simulink model "heli"  (R2023b)
settings: Solver=FixedStepAuto  StartTime=0  StopTime=Ts  FixedStep=0.0025  MaxStep=0.01  RelTol=1e-3  AbsTol=1e-3
undefined symbols (not defined in the file): h, I, ic_euler_ang
libraries: simulink_extras x12, matrix_library x9, AP_Conector x2, shared6dof x1, aerolibobsolete x1
settings Model: Creator=FlightSim2  LastModifiedBy=okmatteson
settings SolverCC: AutoScaleAbsTol=off  AlgebraicLoopSolver=TrustRegion
settings DataIOCC: SaveFormat=Array  SaveOutput=off  SaveTime=off  ReturnWorkspaceOutputs=off
settings OptimizationCC: BlockReduction=off  BooleanDataType=off  ExpressionDepthLimit=2147483647  InitFltsAndDblsToZero=on  LifeSpan=inf
settings DebuggingCC: AlgebraicLoopMsg=none  SaveWithParameterizedLinksMsg=none  MergeDetectMultiDrivingBlocksExec=none  SignalResolutionControl=TryResolveAllWithWarning  InheritedTsInSrcMsg=none  MultiTaskDSMMsg=warning  MultiTaskCondExecSysMsg=none  FcnCallInpInsideContextMsg=warning  AllowSymbolicDim=off  UnknownTsInhSupMsg=none  StateNameClashWarn=warning  SFUnexpectedBacktrackingDiag=warning  SFNoUnconditionalDefaultTransitionDiag=warning  SFExecutionAtInitializationDiag=none  ArithmeticOperatorsInVariantConditions=warning
settings HardwareCC: ProdBitPerPointer=32  ProdBitPerSizeT=32  ProdBitPerPtrDiffT=32  ProdLargestAtomicFloat=None  ProdIntDivRoundTo=Undefined  ProdEndianess=Unspecified  ProdWordSize=32  ProdHWDeviceType=32-bit Generic  TargetUnknown=on
settings ModelReferenceCC: EnableRefExpFcnMdlSchedulingChecks=on  PropagateSignalLabelsOutOfModel=off
settings SFSimCC: SimUseLocalCustomCode=off  CustomCodeUndefinedFunction=UseInterfaceOnly
settings RTWCC: TemplateMakefile=grt_unix.tmf  RTWUseLocalCustomCode=off
settings CodeAppCC: StateflowObjectComments=on
settings GRTTargetCC: TargetFcnLib=ansi_tfl_tmw.mat  TargetLangStandard=C89/C90 (ANSI)  CombineOutputUpdateFcns=off  GRTInterface=on
settings ConfigComp: CovMetricSettings=dw  CovSaveCumulativeToWorkspaceVar=on  CovSaveSingleToWorkspaceVar=on  CovExternalEMLEnable=off

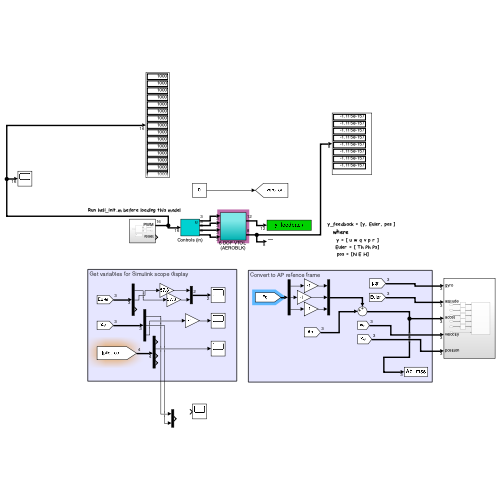
[thumbnail: Simulink's stored preview of the top-level diagram]
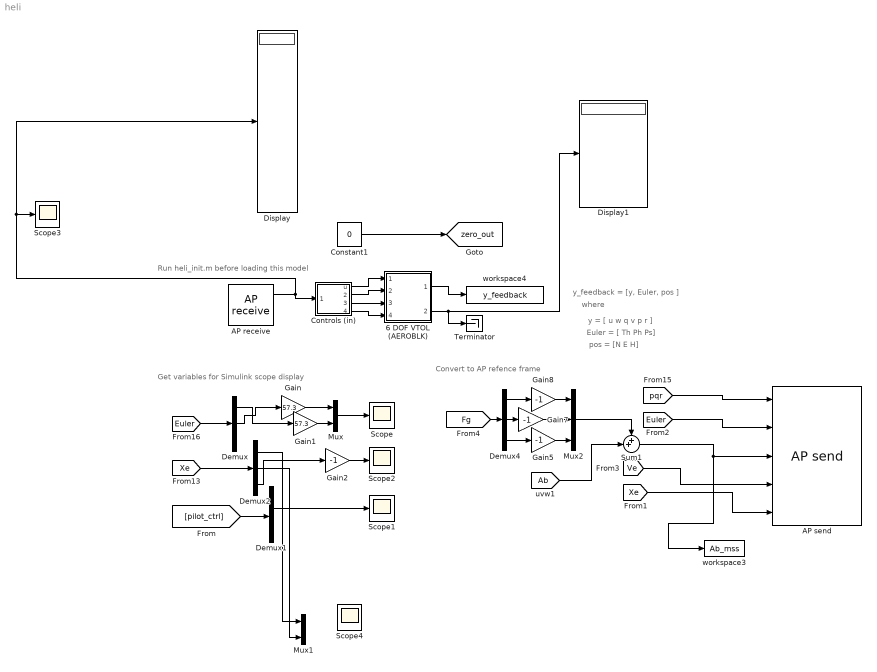
== system heli ==
  note: Run heli_init.m before loading this model
  note: Convert to AP refence frame
  note: Get variables for Simulink scope display
  note: y_feedback = [y, Euler, pos ]
  note: pos = [N E H]
  note: Euler = [ Th Ph Ps]
  note: y = [ u w q v p r ]
  note: where
  6 DOF VTOL (AEROBLK) : Subsystem
  AP receive : AP_Conector/AP receive  SystemSampleTime=-1  VariantActivationTime=update diagram  AllowFlexibleInterface=on  Latency=0  AutoFrameSizeCalculation=off
  AP send : AP_Conector/AP send  SystemSampleTime=-1  VariantActivationTime=update diagram  AllowFlexibleInterface=on  Latency=0  AutoFrameSizeCalculation=off
  Constant1 : Constant  Value=0
  Controls (in) : Subsystem
      mask Display: port_label('output',1,'u','texmode','on');
  Demux : Demux  Outputs=3
  Demux1 : Demux
  Demux2 : Demux  Outputs=3
  Demux4 : Demux  Outputs=3
  Display : Display
  Display1 : Display
  Gain : Gain  Gain=57.3
  Gain1 : Gain  Gain=57.3
  Gain{2,5,7..8} (4 alike) : Gain  Gain=-1
  Mux : Mux  Inputs=2
  Mux1 : Mux  Inputs=2
  Mux2 : Mux  Inputs=3
  Scope{,1..4} (5 alike) : Scope
  Sum1 : Sum  Inputs=++|
  Terminator : Terminator
  workspace3 : ToWorkspace  VariableName=Ab_mss
      settings: MaxDataPoints=max_saved
  workspace4 : ToWorkspace  VariableName=y_feedback
      settings: MaxDataPoints=max_saved
  tag scope: zero_out=global
  wires:
  Controls (in)/1(u) -> 6 DOF VTOL (AEROBLK)/1(Control1)
  6 DOF VTOL (AEROBLK)/1(Out1) -> workspace4/1
  [Euler] -> Demux/1
  Demux/1 -> Gain1/1
  Demux/2 -> Gain/1
  Mux/1 -> Scope/1
  [pilot_ctrl] -> Demux1/1
  Demux1/2 -> Scope1/1
  [Xe] -> Demux2/1
  Demux2/3 -> Gain2/1
  Gain/1 -> Mux/1
  Gain1/1 -> Mux/2
  Gain2/1 -> Scope2/1
  [pqr] -> AP send/1
  [Euler] -> AP send/2
  [Ve] -> AP send/4
  [Xe] -> AP send/5
  [Ab] -> Sum1/2
  [Fg] -> Demux4/1
  Demux4/1 -> Gain8/1
  Demux4/2 -> Gain7/1
  Mux2/1 -> Sum1/1
  Gain5/1 -> Mux2/3
  Demux4/3 -> Gain5/1
  Sum1/1 -> workspace3/1, AP send/3
  Gain8/1 -> Mux2/1
  Gain7/1 -> Mux2/2
  Constant1/1 -> [zero_out]
  Controls (in)/2(Outport) -> 6 DOF VTOL (AEROBLK)/2(Input)
  Controls (in)/3(Outport1) -> 6 DOF VTOL (AEROBLK)/3(Input1)
  Controls (in)/4(Outport2) -> 6 DOF VTOL (AEROBLK)/4(Input2)
  AP receive/1 -> Controls (in)/1(In1), Scope3/1, Display/1
  6 DOF VTOL (AEROBLK)/2(Outport) -> Terminator/1, Display1/1
  Demux2/1 -> Mux1/1
  Demux2/2 -> Mux1/2

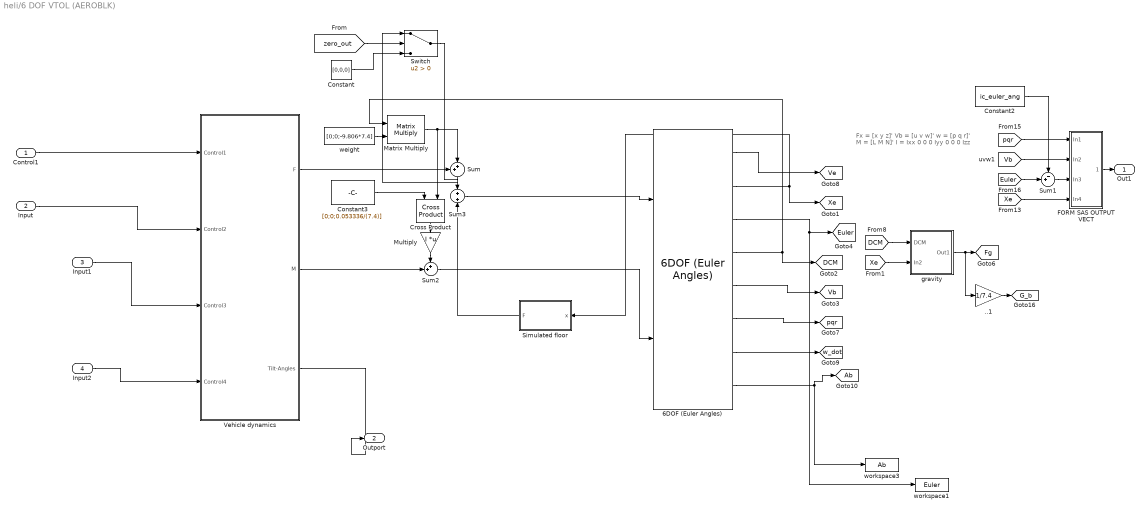
== system heli/6 DOF VTOL (AEROBLK) ==
  note: Fx = [x y z]'
      |
      | Vb = [u v w]'
      |
      | w = [p q r]'
      |
      | M = [L M N]'
      |
      | I =  Ixx  0     0
      |      0   Iyy    0
      |        	  0   0    Izz
  Control1 : Inport
  Input : Inport  Port=2
  Input1 : Inport  Port=3
  Input2 : Inport  Port=4
  ..1 : Gain  Gain=1/7.4  SaturateOnIntegerOverflow=on  OutDataTypeStr=Inherit: Same as input  ParamDataTypeStr=Inherit: Same as input
  6DOF (Euler Angles) : shared6dof/6DOF (Euler Angles)  units=Metric (MKS)  mtype=Fixed  rep=Euler Angles  xme_0=[0 0 0]  Vm_0=[0 0 0]  eul_0=[0 0 0]  pm_0=[0 0 0]  mass_0=7.4  mass_e=0.5  mass_f=2.0  inertia=I  inertia_e=eye(3)  inertia_f=2*eye(3)  k_quat=1.0  vre_flag=on  abi_flag=off  aMode=0  xme_statename=''  Vm_statename=''  eul_statename=''  quat_statename=''  pm_statename=''  mass_statename=''
  Constant : Constant  Value=[0,0,0]
  Constant2 : Constant  Value=ic_euler_ang
  Constant3 : Constant  Value=[0;0;0.053336/(7.4)]
  Cross Product : matrix_library/Cross Product
  FORM SAS OUTPUT VECT : Subsystem
      mask Display:
      | port_label('input',1,'pqr','texmode','on');
      | port_label('input',2,'Vb','texmode','on');
      | port_label('input',3,'Euler','texmode','on');
      | port_label('input',4,'Xe','texmode','on');
      | port_label('output',1,'y','texmode','on');
  Matrix Multiply : Product  Multiplication=Matrix(*)
  Multiply : Gain  Gain=I  Multiplication=Matrix(K*u)
  Simulated floor : MATLAB Function  TreatAsAtomicUnit=on  mask{x1=[-100; -0.1], x2=[100; -0.1], E=1000000, thickness=0.1, A=0.5^2}
  Sum : Sum  Inputs=++|
  Sum1 : Sum  Inputs=-+|
  Sum2 : Sum  Inputs=++|
  Sum3 : Sum  Inputs=+|+
  Switch : Switch  Criteria=u2 > Threshold  SaturateOnIntegerOverflow=off  InputSameDT=off
  Vehicle dynamics : Subsystem
  gravity : Subsystem
      mask Display:
      | port_label('input',1,'DCM','texmode','on');
      | port_label('input',2,'Xe','texmode','on');
      | port_label('output',1,'Fg','texmode','on');
  weight : Constant  Value=[0;0;-9.806*7.4]
  workspace1 : ToWorkspace  VariableName=Euler
      settings: MaxDataPoints=max_saved
  workspace3 : ToWorkspace  VariableName=Ab
      settings: MaxDataPoints=max_saved
  Out1 : Outport  VectorParamsAs1DForOutWhenUnconnected=off
  Outport : Outport  Port=2
  tag scope: Ab=global, DCM=global, Euler=global, Fg=global, G_b=global, Vb=global, Ve=global, Xe=global, pqr=global, w_dot=global
  wires:
  Control1/1 -> Vehicle dynamics/1(Control1)
  [pqr] -> FORM SAS OUTPUT VECT/1(In1)
  [Vb] -> FORM SAS OUTPUT VECT/2(In2)
  [Xe] -> FORM SAS OUTPUT VECT/4(In4)
  FORM SAS OUTPUT VECT/1(Out1) -> Out1/1
  6DOF (Euler Angles)/1 -> [Ve]
  6DOF (Euler Angles)/2 -> [Xe], Simulated floor/1(x)
  6DOF (Euler Angles)/4 -> [DCM], Matrix Multiply/1
  6DOF (Euler Angles)/5 -> [Vb]
  6DOF (Euler Angles)/6 -> [pqr]
  6DOF (Euler Angles)/7 -> [w_dot]
  6DOF (Euler Angles)/8 -> [Ab], workspace3/1
  Sum1/1 -> FORM SAS OUTPUT VECT/3(In3)
  gravity/1(Out1) -> ..1/1, [Fg]
  [Xe] -> gravity/2(In2)
  [DCM] -> gravity/1(DCM)
  ..1/1 -> [G_b]
  Constant2/1 -> Sum1/1
  [Euler] -> Sum1/2
  Input/1 -> Vehicle dynamics/2(Control2)
  Input1/1 -> Vehicle dynamics/3(Control3)
  Input2/1 -> Vehicle dynamics/4(Control4)
  Multiply/1 -> Sum2/1
  Cross Product/1 -> Multiply/1
  Vehicle dynamics/2(M) -> Sum2/2
  Constant3/1 -> Cross Product/1
  Sum2/1 -> 6DOF (Euler Angles)/2
  Sum3/1 -> 6DOF (Euler Angles)/1
  Matrix Multiply/1 -> Cross Product/2, Sum/2
  weight/1 -> Matrix Multiply/2
  6DOF (Euler Angles)/3 -> workspace1/1, [Euler]
  Simulated floor/1(F) -> Sum3/2
  Vehicle dynamics/1(F) -> Sum/1
  Switch/1 -> Sum3/1
  Constant/1 -> Switch/3
  Sum/1 -> Switch/1
  [zero_out] -> Switch/2
  Vehicle dynamics/3(Tilt-Angles) -> Outport/1

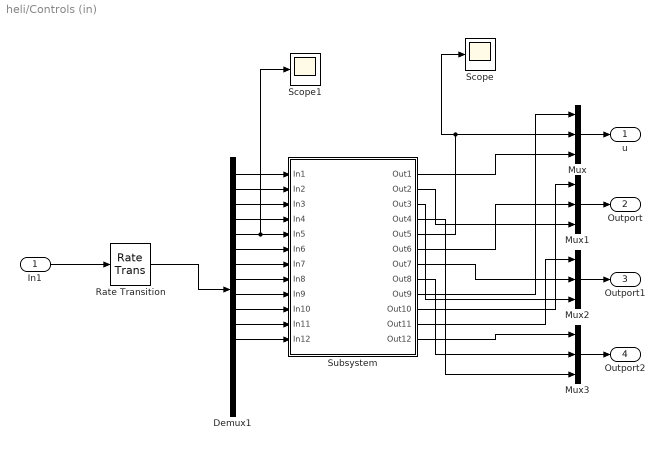
== system heli/Controls (in) ==
  In1 : Inport
  Demux1 : Demux  Outputs=16
  Mux{,1..3} (4 alike) : Mux  Inputs=3
  Rate Transition : RateTransition
  Scope : Scope
  Scope1 : Scope
  Subsystem : Subsystem
  u : Outport  VectorParamsAs1DForOutWhenUnconnected=off
  Outport : Outport  Port=2
  Outport1 : Outport  Port=3
  Outport2 : Outport  Port=4
  wires:
  In1/1 -> Rate Transition/1
  Subsystem/1(Out1) -> Mux/3
  Rate Transition/1 -> Demux1/1
  Demux1/2 -> Subsystem/2(In2)
  Demux1/7 -> Subsystem/7(In7)
  Subsystem/9(Out9) -> Mux/1
  Mux/1 -> u/1
  Demux1/12 -> Subsystem/12(In12)
  Demux1/10 -> Subsystem/10(In10)
  Subsystem/6(Out6) -> Mux1/2
  Demux1/6 -> Subsystem/6(In6)
  Subsystem/12(Out12) -> Mux3/1
  Subsystem/2(Out2) -> Mux1/3
  Subsystem/10(Out10) -> Mux1/1
  Subsystem/11(Out11) -> Mux2/1
  Demux1/9 -> Subsystem/9(In9)
  Subsystem/4(Out4) -> Mux3/3
  Mux1/1 -> Outport/1
  Subsystem/8(Out8) -> Mux3/2
  Subsystem/5(Out5) -> Mux/2, Scope/1
  Demux1/4 -> Subsystem/4(In4)
  Subsystem/7(Out7) -> Mux2/2
  Mux2/1 -> Outport1/1
  Mux3/1 -> Outport2/1
  Demux1/11 -> Subsystem/11(In11)
  Demux1/5 -> Scope1/1, Subsystem/5(In5)
  Demux1/8 -> Subsystem/8(In8)
  Subsystem/3(Out3) -> Mux2/3
  Demux1/1 -> Subsystem/1(In1)
  Demux1/3 -> Subsystem/3(In3)

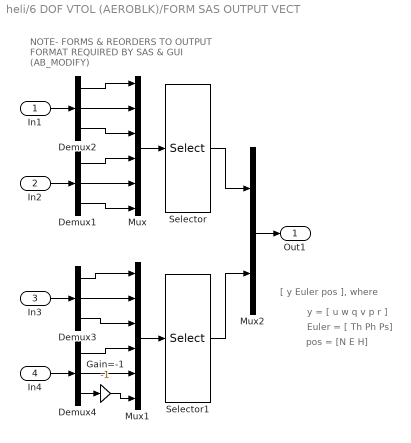
== system heli/6 DOF VTOL (AEROBLK)/FORM SAS OUTPUT VECT ==
  note: NOTE- FORMS & REORDERS TO OUTPUT FORMAT
      | REQUIRED BY SAS & GUI (AB_MODIFY)
  note: [ y Euler pos ], where
  note: pos = [N E H]
  note: Euler = [ Th Ph Ps]
  note: y = [ u w q v p r ]
  In1 : Inport
  In2 : Inport  Port=2
  In3 : Inport  Port=3
  In4 : Inport  Port=4
  Demux{1..4} (4 alike) : Demux  Outputs=3
  Gain=-1 : Gain  Gain=-1
  Mux : Mux  Inputs=6
  Mux1 : Mux  Inputs=6
  Mux2 : Mux  Inputs=2
  Selector : Selector  InputPortWidth=6  IndexOptions=Index vector (dialog)  Indices=[4 6 2 5 1 3]  OutputSizes=1
  Selector1 : Selector  InputPortWidth=6  IndexOptions=Index vector (dialog)  Indices=[2 1 3 4 5 6]  OutputSizes=1
  Out1 : Outport  VectorParamsAs1DForOutWhenUnconnected=off
  wires:
  Demux2/1 -> Mux/1
  Demux2/2 -> Mux/2
  Demux1/1 -> Mux/4
  Demux1/2 -> Mux/5
  Demux1/3 -> Mux/6
  Mux/1 -> Selector/1
  Demux2/3 -> Mux/3
  Mux1/1 -> Selector1/1
  Selector/1 -> Mux2/1
  Selector1/1 -> Mux2/2
  Demux3/1 -> Mux1/1
  Demux3/2 -> Mux1/2
  Demux3/3 -> Mux1/3
  Demux4/1 -> Mux1/4
  Demux4/2 -> Mux1/5
  Gain=-1/1 -> Mux1/6
  Demux4/3 -> Gain=-1/1
  In1/1 -> Demux2/1
  In2/1 -> Demux1/1
  Mux2/1 -> Out1/1
  In3/1 -> Demux3/1
  In4/1 -> Demux4/1

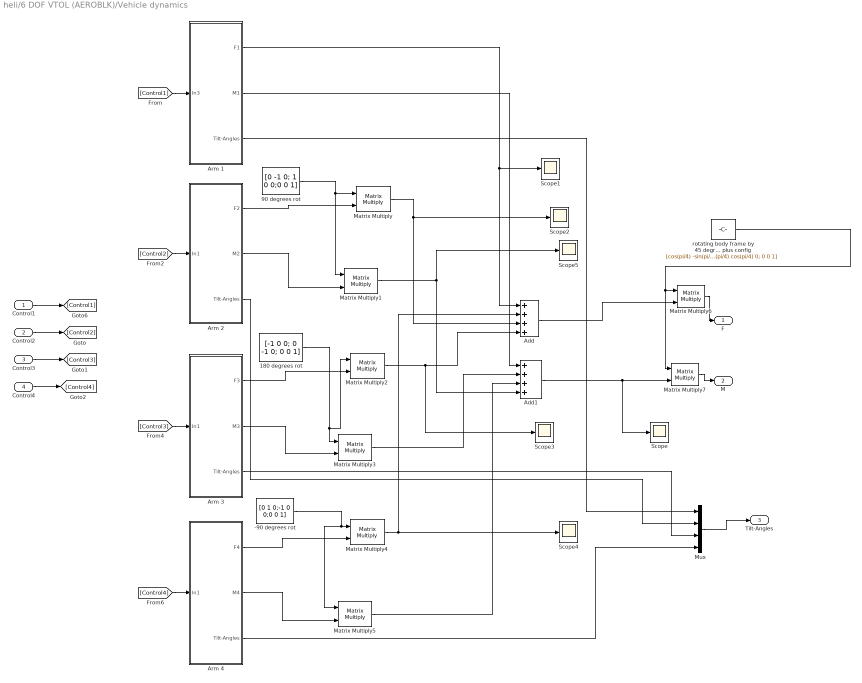
== system heli/6 DOF VTOL (AEROBLK)/Vehicle dynamics ==
  Control1 : Inport
  Control2 : Inport  Port=2
  Control3 : Inport  Port=3
  Control4 : Inport  Port=4
  -90 degrees rot : Constant  Value=[0 1 0;-1 0 0;0 0 1]
  180 degrees rot : Constant  Value=[-1 0 0; 0 -1 0; 0 0 1]
  90 degrees rot : Constant  Value=[0 -1 0; 1 0 0;0 0 1]
  Add : Sum  Inputs=++++
  Add1 : Sum  Inputs=++++
  Arm 1 : Subsystem
  Arm 2 : Subsystem
  Arm 3 : Subsystem
  Arm 4 : Subsystem
  Matrix Multiply{,1..7} (8 alike) : Product  Multiplication=Matrix(*)
  Mux : Mux
  Scope{,1..5} (6 alike) : Scope
  rotating body frame by 45 degrees to X config because vehicle dynamics was done in plus config : Constant  Value=|
      | [cos(pi/4) -sin(pi/4) 0;
      | sin(pi/4) cos(pi/4) 0;
      | 0 0 1]
  F : Outport
  M : Outport  Port=2
  Tilt-Angles : Outport  Port=3
  wires:
  Control1/1 -> [Control1]
  Control2/1 -> [Control2]
  Control3/1 -> [Control3]
  Control4/1 -> [Control4]
  [Control1] -> Arm 1/1(In3)
  Arm 1/1(F1) -> Add/1, Scope1/1
  Arm 1/2(M1) -> Add1/1
  90 degrees rot/1 -> Matrix Multiply1/1, Matrix Multiply/1
  Arm 2/1(F2) -> Matrix Multiply/2
  Matrix Multiply/1 -> Scope2/1, Add/3
  Arm 2/2(M2) -> Matrix Multiply1/2
  Matrix Multiply1/1 -> Add1/4, Scope5/1
  [Control2] -> Arm 2/1(In1)
  -90 degrees rot/1 -> Matrix Multiply5/1, Matrix Multiply4/1
  Arm 3/1(F3) -> Matrix Multiply2/2
  Matrix Multiply3/1 -> Add1/2
  [Control3] -> Arm 3/1(In1)
  Arm 3/2(M3) -> Matrix Multiply3/2
  180 degrees rot/1 -> Matrix Multiply3/1, Matrix Multiply2/1
  Arm 4/2(M4) -> Matrix Multiply5/2
  Arm 4/1(F4) -> Matrix Multiply4/2
  Matrix Multiply5/1 -> Add1/3
  [Control4] -> Arm 4/1(In1)
  Matrix Multiply2/1 -> Scope3/1, Add/4
  Matrix Multiply4/1 -> Add/2, Scope4/1
  rotating body frame by 45 degrees to X config because vehicle dynamics was done in plus config/1 -> Matrix Multiply6/1, Matrix Multiply7/1
  Add/1 -> Matrix Multiply6/2
  Add1/1 -> Matrix Multiply7/2, Scope/1
  Matrix Multiply7/1 -> M/1
  Matrix Multiply6/1 -> F/1
  Arm 1/3(Tilt-Angles) -> Mux/1
  Arm 2/3(Tilt-Angles) -> Mux/2
  Arm 3/3(Tilt-Angles) -> Mux/3
  Arm 4/3(Tilt-Angles) -> Mux/4
  Mux/1 -> Tilt-Angles/1

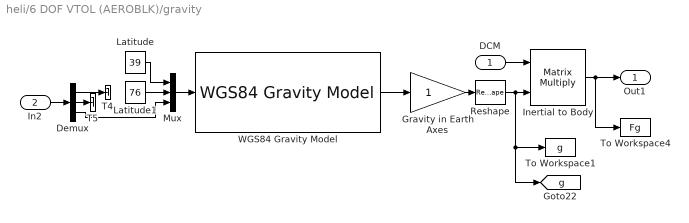
== system heli/6 DOF VTOL (AEROBLK)/gravity ==
  DCM : Inport
  In2 : Inport  Port=2
  Demux : Demux  Outputs=3
  Gravity in Earth Axes : Gain  SaturateOnIntegerOverflow=on  OutDataTypeStr=Inherit: Same as input  ParamDataTypeStr=Inherit: Same as input
  Inertial to Body : Product  Multiplication=Matrix(*)  InputSameDT=on  SaturateOnIntegerOverflow=on  OutDataTypeStr=Inherit: Same as first input
  Latitude : Constant  Value=39
  Latitude1 : Constant  Value=76
  Mux : Mux  Inputs=3
  Reshape : Reshape
  T4 : Terminator
  T5 : Terminator
  To Workspace1 : ToWorkspace  VariableName=g  SampleTime=-1
      settings: MaxDataPoints=max_saved
  To Workspace4 : ToWorkspace  VariableName=Fg  SampleTime=-1
      settings: MaxDataPoints=max_saved
  "WGS84 Gravity Model " : aerolibobsolete/WGS84 Gravity Model   model=WGS84 Exact  units=Metric (MKS)  no_atmos=on  precessing=on  jd_loc=off  month=October  day=10  year=2004  no_centrifugal=on  action=None
  Out1 : Outport  VectorParamsAs1DForOutWhenUnconnected=off
  tag scope: g=global
  wires:
  In2/1 -> Demux/1
  Demux/2 -> T5/1
  Demux/1 -> T4/1
  Inertial to Body/1 -> To Workspace4/1, Out1/1
  DCM/1 -> Inertial to Body/1
  Gravity in Earth Axes/1 -> Reshape/1
  "WGS84 Gravity Model "/1 -> Gravity in Earth Axes/1
  Mux/1 -> "WGS84 Gravity Model "/1
  Reshape/1 -> Inertial to Body/2, To Workspace1/1, [g]
  Latitude1/1 -> Mux/2
  Latitude/1 -> Mux/1
  Demux/3 -> Mux/3

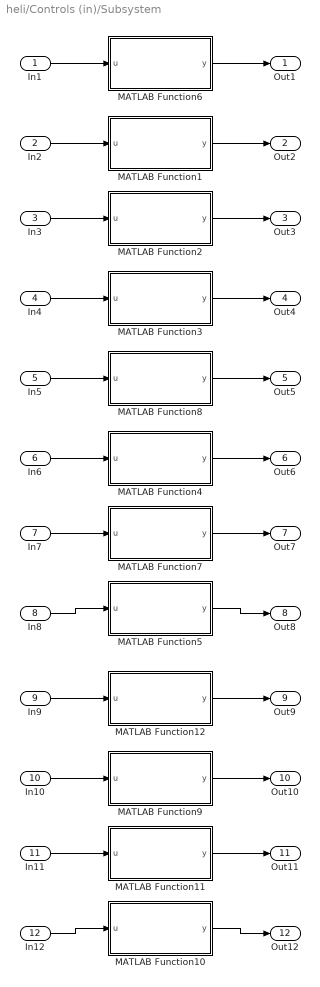
== system heli/Controls (in)/Subsystem ==
  In1 : Inport
  In2 : Inport  Port=2
  In3 : Inport  Port=3
  In4 : Inport  Port=4
  In5 : Inport  Port=5
  In6 : Inport  Port=6
  In7 : Inport  Port=7
  In8 : Inport  Port=8
  In9 : Inport  Port=9
  In10 : Inport  Port=10
  In11 : Inport  Port=11
  In12 : Inport  Port=12
  MATLAB Function1 : MATLAB Function  TreatAsAtomicUnit=on  mask{min_in=1000, min_out=0, max_in=2000, max_out=633}
  MATLAB Function10 : MATLAB Function  TreatAsAtomicUnit=on  mask{min_in=682, min_out=-1.57, max_in=2318, max_out=1.57}
  MATLAB Function11 : MATLAB Function  TreatAsAtomicUnit=on  mask{min_in=682, min_out=-1.57, max_in=2318, max_out=1.57}
  MATLAB Function12 : MATLAB Function  TreatAsAtomicUnit=on  mask{min_in=682, min_out=-1.57, max_in=2318, max_out=1.57}
  MATLAB Function2 : MATLAB Function  TreatAsAtomicUnit=on  mask{min_in=1000, min_out=0, max_in=2000, max_out=633}
  MATLAB Function3 : MATLAB Function  TreatAsAtomicUnit=on  mask{min_in=1000, min_out=0, max_in=2000, max_out=633}
  MATLAB Function4 : MATLAB Function  TreatAsAtomicUnit=on  mask{min_in=682, min_out=-1.57, max_in=2318, max_out=1.57}
  MATLAB Function5 : MATLAB Function  TreatAsAtomicUnit=on  mask{min_in=682, min_out=-1.57, max_in=2318, max_out=1.57}
  MATLAB Function6 : MATLAB Function  TreatAsAtomicUnit=on  mask{min_in=1000, min_out=0, max_in=2000, max_out=633}
  MATLAB Function7 : MATLAB Function  TreatAsAtomicUnit=on  mask{min_in=682, min_out=-1.57, max_in=2318, max_out=1.57}
  MATLAB Function8 : MATLAB Function  TreatAsAtomicUnit=on  mask{min_in=682, min_out=-1.57, max_in=2318, max_out=1.57}
  MATLAB Function9 : MATLAB Function  TreatAsAtomicUnit=on  mask{min_in=682, min_out=-1.57, max_in=2318, max_out=1.57}
  Out1 : Outport
  Out2 : Outport  Port=2
  Out3 : Outport  Port=3
  Out4 : Outport  Port=4
  Out5 : Outport  Port=5
  Out6 : Outport  Port=6
  Out7 : Outport  Port=7
  Out8 : Outport  Port=8
  Out9 : Outport  Port=9
  Out10 : Outport  Port=10
  Out11 : Outport  Port=11
  Out12 : Outport  Port=12
  wires:
  In1/1 -> MATLAB Function6/1(u)
  MATLAB Function6/1(y) -> Out1/1
  In2/1 -> MATLAB Function1/1(u)
  MATLAB Function1/1(y) -> Out2/1
  MATLAB Function2/1(y) -> Out3/1
  In3/1 -> MATLAB Function2/1(u)
  In4/1 -> MATLAB Function3/1(u)
  MATLAB Function3/1(y) -> Out4/1
  In5/1 -> MATLAB Function8/1(u)
  MATLAB Function8/1(y) -> Out5/1
  MATLAB Function4/1(y) -> Out6/1
  In6/1 -> MATLAB Function4/1(u)
  In7/1 -> MATLAB Function7/1(u)
  MATLAB Function7/1(y) -> Out7/1
  In8/1 -> MATLAB Function5/1(u)
  MATLAB Function5/1(y) -> Out8/1
  In9/1 -> MATLAB Function12/1(u)
  MATLAB Function12/1(y) -> Out9/1
  MATLAB Function9/1(y) -> Out10/1
  In10/1 -> MATLAB Function9/1(u)
  In11/1 -> MATLAB Function11/1(u)
  MATLAB Function11/1(y) -> Out11/1
  In12/1 -> MATLAB Function10/1(u)
  MATLAB Function10/1(y) -> Out12/1

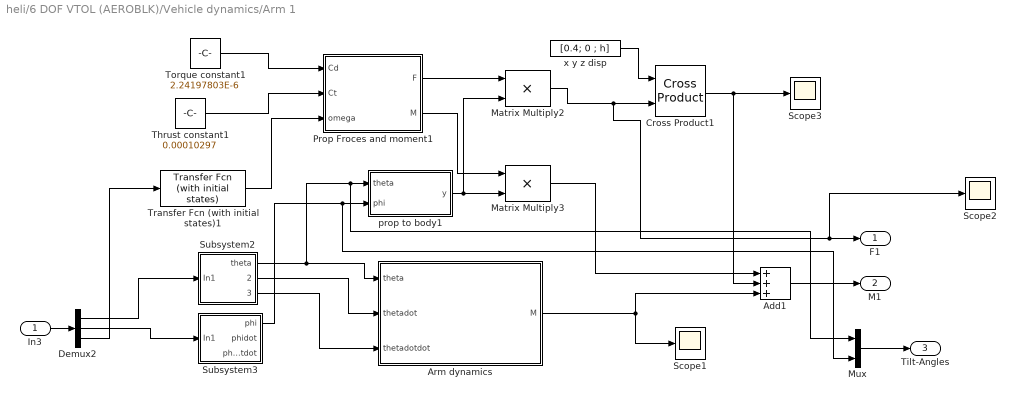
== system heli/6 DOF VTOL (AEROBLK)/Vehicle dynamics/Arm 1 ==
  In3 : Inport
  Add1 : Sum  Inputs=+++
  Arm dynamics : Subsystem
  Cross Product1 : matrix_library/Cross Product
  Demux2 : Demux  Outputs=3
  Matrix Multiply2 : Product
  Matrix Multiply3 : Product
  Mux : Mux  Inputs=2
  Prop Froces and moment1 : Subsystem
  Scope1 : Scope
  Scope2 : Scope
  Scope3 : Scope
  Subsystem2 : Subsystem
  Subsystem3 : Subsystem
  Thrust constant1 : Constant  Value=0.00010297
  Torque constant1 : Constant  Value=2.24197803E-6
  Transfer Fcn (with initial states)1 : simulink_extras/Additional Linear/Transfer Fcn (with initial states)  N=[153.35]  D=[1 20.06 153.35]  X0=0
  prop to body1 : MATLAB Function  TreatAsAtomicUnit=on
  x y z disp : Constant  Value=[0.4; 0 ; h]
  F1 : Outport
  M1 : Outport  Port=2
  Tilt-Angles : Outport  Port=3
  wires:
  x y z disp/1 -> Cross Product1/1
  Subsystem2/2(thetadot) -> Arm dynamics/2(thetadot)
  Cross Product1/1 -> Add1/2, Scope3/1
  In3/1 -> Demux2/1
  Prop Froces and moment1/1(F) -> Matrix Multiply2/1
  Arm dynamics/1(M) -> Add1/3, Scope1/1
  Demux2/2 -> Subsystem3/1(In1)
  Thrust constant1/1 -> Prop Froces and moment1/2(Ct)
  Torque constant1/1 -> Prop Froces and moment1/1(Cd)
  Add1/1 -> M1/1
  Matrix Multiply3/1 -> Add1/1
  prop to body1/1(y) -> Matrix Multiply3/2, Matrix Multiply2/2
  Prop Froces and moment1/2(M) -> Matrix Multiply3/1
  Demux2/1 -> Subsystem2/1(In1)
  Subsystem2/1(theta) -> Arm dynamics/1(theta), Mux/1, prop to body1/1(theta)
  Matrix Multiply2/1 -> Cross Product1/2, Scope2/1, F1/1
  Subsystem3/1(phi) -> Mux/2, prop to body1/2(phi)
  Subsystem2/3(thetadotdot) -> Arm dynamics/3(thetadotdot)
  Demux2/3 -> Transfer Fcn (with initial states)1/1
  Transfer Fcn (with initial states)1/1 -> Prop Froces and moment1/3(omega)
  Mux/1 -> Tilt-Angles/1

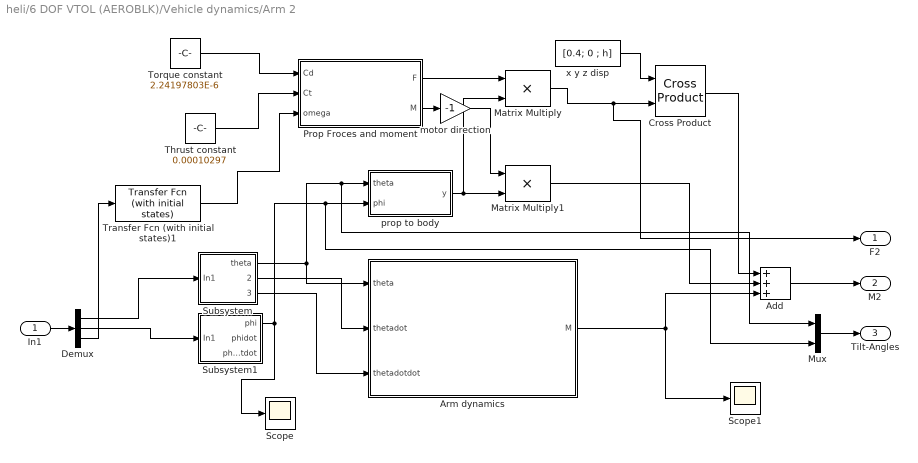
== system heli/6 DOF VTOL (AEROBLK)/Vehicle dynamics/Arm 2 ==
  In1 : Inport
  Add : Sum  Inputs=+++
  Arm dynamics : Subsystem
  Cross Product : matrix_library/Cross Product
  Demux : Demux  Outputs=3
  Matrix Multiply : Product
  Matrix Multiply1 : Product
  Mux : Mux  Inputs=2
  Prop Froces and moment : Subsystem
  Scope : Scope
  Scope1 : Scope
  Subsystem : Subsystem
  Subsystem1 : Subsystem
  Thrust constant : Constant  Value=0.00010297
  Torque constant : Constant  Value=2.24197803E-6
  Transfer Fcn (with initial states)1 : simulink_extras/Additional Linear/Transfer Fcn (with initial states)  N=[153.35]  D=[1 20.06 153.35]  X0=0
  motor direction : Gain  Gain=-1
  prop to body : MATLAB Function  TreatAsAtomicUnit=on
  x y z disp : Constant  Value=[0.4; 0 ; h]
  F2 : Outport
  M2 : Outport  Port=2
  Tilt-Angles : Outport  Port=3
  wires:
  prop to body/1(y) -> Matrix Multiply1/2, Matrix Multiply/2
  Demux/2 -> Subsystem1/1(In1)
  Matrix Multiply/1 -> Cross Product/2, F2/1
  Prop Froces and moment/1(F) -> Matrix Multiply/1
  Subsystem/1(theta) -> Arm dynamics/1(theta), Mux/1, prop to body/1(theta)
  Matrix Multiply1/1 -> Add/2
  Prop Froces and moment/2(M) -> motor direction/1
  Subsystem1/1(phi) -> Scope/1, Mux/2, prop to body/2(phi)
  Demux/1 -> Subsystem/1(In1)
  x y z disp/1 -> Cross Product/1
  Add/1 -> M2/1
  Torque constant/1 -> Prop Froces and moment/1(Cd)
  Thrust constant/1 -> Prop Froces and moment/2(Ct)
  Cross Product/1 -> Add/1
  In1/1 -> Demux/1
  Subsystem/2(thetadot) -> Arm dynamics/2(thetadot)
  Subsystem/3(thetadotdot) -> Arm dynamics/3(thetadotdot)
  Arm dynamics/1(M) -> Add/3, Scope1/1
  Demux/3 -> Transfer Fcn (with initial states)1/1
  motor direction/1 -> Matrix Multiply1/1
  Transfer Fcn (with initial states)1/1 -> Prop Froces and moment/3(omega)
  Mux/1 -> Tilt-Angles/1

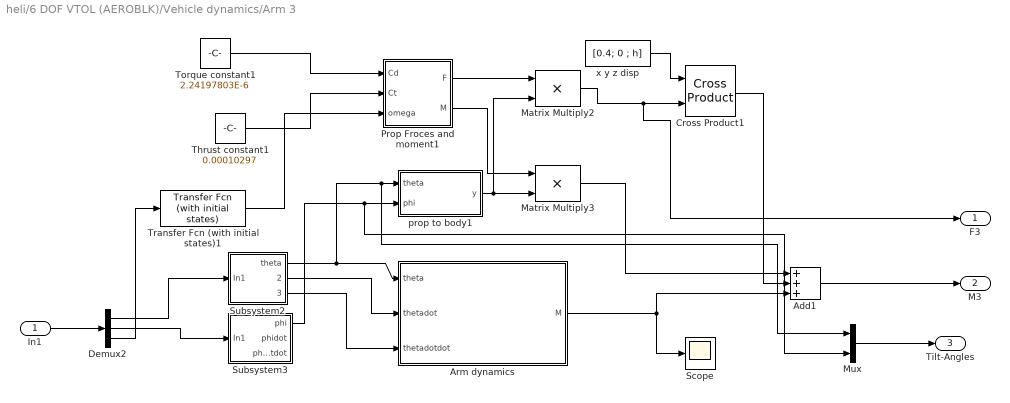
== system heli/6 DOF VTOL (AEROBLK)/Vehicle dynamics/Arm 3 ==
  In1 : Inport
  Add1 : Sum  Inputs=+++
  Arm dynamics : Subsystem
  Cross Product1 : matrix_library/Cross Product
  Demux2 : Demux  Outputs=3
  Matrix Multiply2 : Product
  Matrix Multiply3 : Product
  Mux : Mux  Inputs=2
  Prop Froces and moment1 : Subsystem
  Scope : Scope
  Subsystem2 : Subsystem
  Subsystem3 : Subsystem
  Thrust constant1 : Constant  Value=0.00010297
  Torque constant1 : Constant  Value=2.24197803E-6
  Transfer Fcn (with initial states)1 : simulink_extras/Additional Linear/Transfer Fcn (with initial states)  N=[153.35]  D=[1 20.06 153.35]  X0=0
  prop to body1 : MATLAB Function  TreatAsAtomicUnit=on
  x y z disp : Constant  Value=[0.4; 0 ; h]
  F3 : Outport
  M3 : Outport  Port=2
  Tilt-Angles : Outport  Port=3
  wires:
  x y z disp/1 -> Cross Product1/1
  Subsystem2/2(thetadot) -> Arm dynamics/2(thetadot)
  Cross Product1/1 -> Add1/2
  In1/1 -> Demux2/1
  Prop Froces and moment1/1(F) -> Matrix Multiply2/1
  Arm dynamics/1(M) -> Add1/3, Scope/1
  Demux2/2 -> Subsystem3/1(In1)
  Thrust constant1/1 -> Prop Froces and moment1/2(Ct)
  Torque constant1/1 -> Prop Froces and moment1/1(Cd)
  Add1/1 -> M3/1
  Matrix Multiply3/1 -> Add1/1
  prop to body1/1(y) -> Matrix Multiply3/2, Matrix Multiply2/2
  Prop Froces and moment1/2(M) -> Matrix Multiply3/1
  Demux2/1 -> Subsystem2/1(In1)
  Subsystem2/1(theta) -> Arm dynamics/1(theta), Mux/1, prop to body1/1(theta)
  Demux2/3 -> Transfer Fcn (with initial states)1/1
  Matrix Multiply2/1 -> Cross Product1/2, F3/1
  Subsystem3/1(phi) -> Mux/2, prop to body1/2(phi)
  Subsystem2/3(thetadotdot) -> Arm dynamics/3(thetadotdot)
  Transfer Fcn (with initial states)1/1 -> Prop Froces and moment1/3(omega)
  Mux/1 -> Tilt-Angles/1

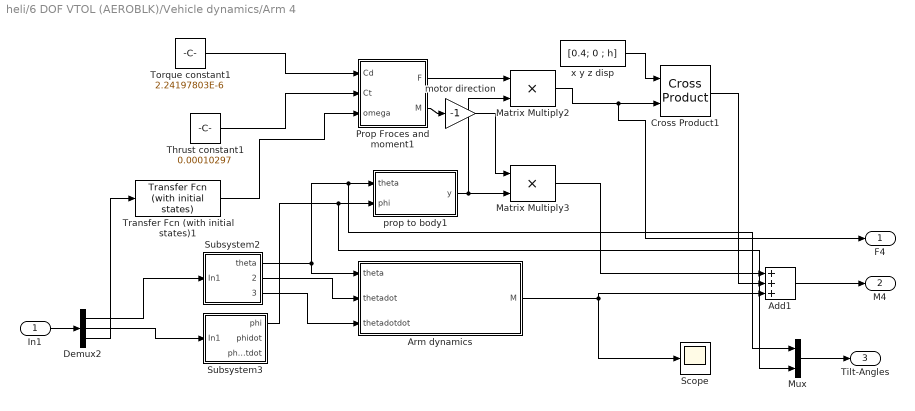
== system heli/6 DOF VTOL (AEROBLK)/Vehicle dynamics/Arm 4 ==
  In1 : Inport
  Add1 : Sum  Inputs=+++
  Arm dynamics : Subsystem
  Cross Product1 : matrix_library/Cross Product
  Demux2 : Demux  Outputs=3
  Matrix Multiply2 : Product
  Matrix Multiply3 : Product
  Mux : Mux  Inputs=2
  Prop Froces and moment1 : Subsystem
  Scope : Scope
  Subsystem2 : Subsystem
  Subsystem3 : Subsystem
  Thrust constant1 : Constant  Value=0.00010297
  Torque constant1 : Constant  Value=2.24197803E-6
  Transfer Fcn (with initial states)1 : simulink_extras/Additional Linear/Transfer Fcn (with initial states)  N=[153.35]  D=[1 20.06 153.35]  X0=0
  motor direction : Gain  Gain=-1
  prop to body1 : MATLAB Function  TreatAsAtomicUnit=on
  x y z disp : Constant  Value=[0.4; 0 ; h]
  F4 : Outport
  M4 : Outport  Port=2
  Tilt-Angles : Outport  Port=3
  wires:
  x y z disp/1 -> Cross Product1/1
  Subsystem2/2(thetadot) -> Arm dynamics/2(thetadot)
  Cross Product1/1 -> Add1/2
  In1/1 -> Demux2/1
  Prop Froces and moment1/1(F) -> Matrix Multiply2/1
  Arm dynamics/1(M) -> Add1/3, Scope/1
  Demux2/2 -> Subsystem3/1(In1)
  Thrust constant1/1 -> Prop Froces and moment1/2(Ct)
  Torque constant1/1 -> Prop Froces and moment1/1(Cd)
  Add1/1 -> M4/1
  Matrix Multiply3/1 -> Add1/1
  prop to body1/1(y) -> Matrix Multiply3/2, Matrix Multiply2/2
  Prop Froces and moment1/2(M) -> motor direction/1
  Demux2/1 -> Subsystem2/1(In1)
  Subsystem2/1(theta) -> Arm dynamics/1(theta), Mux/1, prop to body1/1(theta)
  Matrix Multiply2/1 -> Cross Product1/2, F4/1
  Subsystem3/1(phi) -> Mux/2, prop to body1/2(phi)
  Subsystem2/3(thetadotdot) -> Arm dynamics/3(thetadotdot)
  Demux2/3 -> Transfer Fcn (with initial states)1/1
  motor direction/1 -> Matrix Multiply3/1
  Transfer Fcn (with initial states)1/1 -> Prop Froces and moment1/3(omega)
  Mux/1 -> Tilt-Angles/1

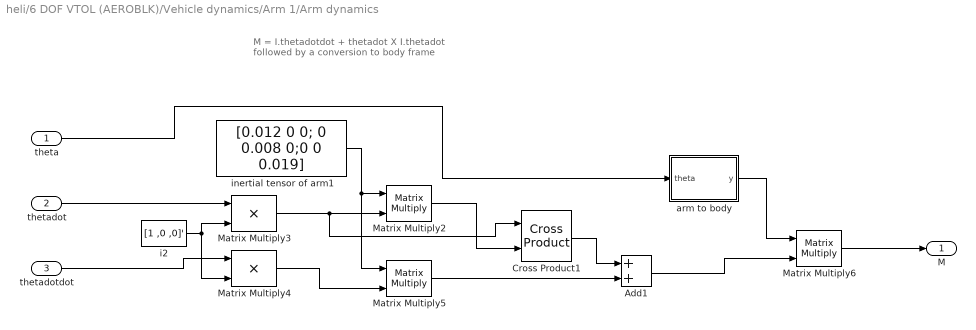
== system heli/6 DOF VTOL (AEROBLK)/Vehicle dynamics/Arm 1/Arm dynamics ==
  note: M = I.thetadotdot + thetadot X I.thetadot
      | followed by a conversion to body frame
  theta : Inport
  thetadot : Inport  Port=2
  thetadotdot : Inport  Port=3
  Add1 : Sum
  Cross Product1 : matrix_library/Cross Product
  Matrix Multiply2 : Product  Multiplication=Matrix(*)
  Matrix Multiply3 : Product
  Matrix Multiply4 : Product
  Matrix Multiply5 : Product  Multiplication=Matrix(*)
  Matrix Multiply6 : Product  Multiplication=Matrix(*)
  arm to body : MATLAB Function  TreatAsAtomicUnit=on
  i2 : Constant  Value=[1 ,0 ,0]'
  inertial tensor of arm1 : Constant  Value=[0.012 0 0; 0 0.008 0;0 0 0.019]
  M : Outport
  wires:
  Matrix Multiply3/1 -> Cross Product1/1, Matrix Multiply2/2
  inertial tensor of arm1/1 -> Matrix Multiply5/1, Matrix Multiply2/1
  thetadotdot/1 -> Matrix Multiply4/1
  Matrix Multiply4/1 -> Matrix Multiply5/2
  Matrix Multiply5/1 -> Add1/2
  i2/1 -> Matrix Multiply4/2, Matrix Multiply3/2
  arm to body/1(y) -> Matrix Multiply6/1
  Matrix Multiply2/1 -> Cross Product1/2
  Cross Product1/1 -> Add1/1
  Add1/1 -> Matrix Multiply6/2
  thetadot/1 -> Matrix Multiply3/1
  Matrix Multiply6/1 -> M/1
  theta/1 -> arm to body/1(theta)

== system heli/6 DOF VTOL (AEROBLK)/Vehicle dynamics/Arm 1/Prop Froces and moment1 ==
  note: T = Ctx w^2
      | Q = Cd x w^2
  Cd : Inport
  Ct : Inport  Port=2
  omega : Inport  Port=3
  Product{,1..3} (4 alike) : Product
  F : Outport
  M : Outport  Port=2
  wires:
  omega/1 -> Product3/1, Product2/2, Product1/2, Product/2
  Ct/1 -> Product2/1
  Product2/1 -> Product3/2
  Product3/1 -> F/1
  Product/1 -> Product1/1
  Product1/1 -> M/1
  Cd/1 -> Product/1

== system heli/6 DOF VTOL (AEROBLK)/Vehicle dynamics/Arm 1/Subsystem2 ==
  In1 : Inport
  Derivative : Derivative
  Derivative1 : Derivative  CoefficientInTFapproximation=1
  Scope : Scope
  Scope1 : Scope
  Scope2 : Scope
  Transfer Fcn (with initial states)1 : simulink_extras/Additional Linear/Transfer Fcn (with initial states)  N=[153.5000]  D="[1  20.06  153.3]"  X0=0
  theta : Outport
  thetadot : Outport  Port=2
  thetadotdot : Outport  Port=3
  wires:
  Derivative/1 -> Scope2/1, thetadot/1, Derivative1/1
  Transfer Fcn (with initial states)1/1 -> Derivative/1, Scope/1, theta/1
  Derivative1/1 -> Scope1/1, thetadotdot/1
  In1/1 -> Transfer Fcn (with initial states)1/1

== system heli/6 DOF VTOL (AEROBLK)/Vehicle dynamics/Arm 1/Subsystem3 ==
  In1 : Inport
  Derivative2 : Derivative
  Derivative3 : Derivative
  Scope : Scope
  Transfer Fcn (with initial states) : simulink_extras/Additional Linear/Transfer Fcn (with initial states)  N=[153.5000]  D="[1  20.06  153.3]"  X0=0
  phi : Outport
  phidot : Outport  Port=2
  phidotdot : Outport  Port=3
  wires:
  Derivative2/1 -> phidot/1, Derivative3/1
  Transfer Fcn (with initial states)/1 -> Derivative2/1, Scope/1, phi/1
  Derivative3/1 -> phidotdot/1
  In1/1 -> Transfer Fcn (with initial states)/1

== system heli/6 DOF VTOL (AEROBLK)/Vehicle dynamics/Arm 2/Arm dynamics ==
  note: M = I.thetadotdot + thetadot X I.thetadot
      | followed by a conversion to body frame
  theta : Inport
  thetadot : Inport  Port=2
  thetadotdot : Inport  Port=3
  Add1 : Sum
  Cross Product1 : matrix_library/Cross Product
  Matrix Multiply2 : Product  Multiplication=Matrix(*)
  Matrix Multiply3 : Product
  Matrix Multiply4 : Product
  Matrix Multiply5 : Product  Multiplication=Matrix(*)
  Matrix Multiply6 : Product  Multiplication=Matrix(*)
  arm to body : MATLAB Function  TreatAsAtomicUnit=on
  i2 : Constant  Value=[1 ,0 ,0]'
  inertial tensor of arm : Constant  Value=[0.012 0 0; 0 0.008 0;0 0 0.019]
  M : Outport
  wires:
  Matrix Multiply3/1 -> Cross Product1/1, Matrix Multiply2/2
  inertial tensor of arm/1 -> Matrix Multiply5/1, Matrix Multiply2/1
  thetadotdot/1 -> Matrix Multiply4/1
  Matrix Multiply4/1 -> Matrix Multiply5/2
  Matrix Multiply5/1 -> Add1/2
  i2/1 -> Matrix Multiply4/2, Matrix Multiply3/2
  arm to body/1(y) -> Matrix Multiply6/1
  Matrix Multiply2/1 -> Cross Product1/2
  Cross Product1/1 -> Add1/1
  Add1/1 -> Matrix Multiply6/2
  thetadot/1 -> Matrix Multiply3/1
  Matrix Multiply6/1 -> M/1
  theta/1 -> arm to body/1(theta)

== system heli/6 DOF VTOL (AEROBLK)/Vehicle dynamics/Arm 2/Prop Froces and moment ==
  note: T = Ctx w^2
      | Q = Cd x w^2
  Cd : Inport
  Ct : Inport  Port=2
  omega : Inport  Port=3
  Product{,1..3} (4 alike) : Product
  F : Outport
  M : Outport  Port=2
  wires:
  omega/1 -> Product3/1, Product2/2, Product1/2, Product/2
  Ct/1 -> Product2/1
  Product2/1 -> Product3/2
  Product3/1 -> F/1
  Product/1 -> Product1/1
  Product1/1 -> M/1
  Cd/1 -> Product/1

== system heli/6 DOF VTOL (AEROBLK)/Vehicle dynamics/Arm 2/Subsystem ==
  In1 : Inport
  Derivative : Derivative
  Derivative1 : Derivative
  Scope : Scope
  Transfer Fcn (with initial states)1 : simulink_extras/Additional Linear/Transfer Fcn (with initial states)  N=[153.5000]  D="[1  20.06  153.3]"  X0=0
  theta : Outport
  thetadot : Outport  Port=2
  thetadotdot : Outport  Port=3
  wires:
  Derivative/1 -> thetadot/1, Derivative1/1
  Transfer Fcn (with initial states)1/1 -> Derivative/1, Scope/1, theta/1
  Derivative1/1 -> thetadotdot/1
  In1/1 -> Transfer Fcn (with initial states)1/1

== system heli/6 DOF VTOL (AEROBLK)/Vehicle dynamics/Arm 2/Subsystem1 ==
  In1 : Inport
  Derivative2 : Derivative
  Derivative3 : Derivative
  Scope : Scope
  Transfer Fcn (with initial states) : simulink_extras/Additional Linear/Transfer Fcn (with initial states)  N=[153.5000]  D="[1  20.06  153.3]"  X0=0
  phi : Outport
  phidot : Outport  Port=2
  phidotdot : Outport  Port=3
  wires:
  Derivative2/1 -> phidot/1, Derivative3/1
  Transfer Fcn (with initial states)/1 -> Derivative2/1, Scope/1, phi/1
  Derivative3/1 -> phidotdot/1
  In1/1 -> Transfer Fcn (with initial states)/1

== system heli/6 DOF VTOL (AEROBLK)/Vehicle dynamics/Arm 3/Arm dynamics ==
  note: M = I.thetadotdot + thetadot X I.thetadot
      | followed by a conversion to body frame
  theta : Inport
  thetadot : Inport  Port=2
  thetadotdot : Inport  Port=3
  Add1 : Sum
  Cross Product1 : matrix_library/Cross Product
  Matrix Multiply2 : Product  Multiplication=Matrix(*)
  Matrix Multiply3 : Product
  Matrix Multiply4 : Product
  Matrix Multiply5 : Product  Multiplication=Matrix(*)
  Matrix Multiply6 : Product  Multiplication=Matrix(*)
  arm to body : MATLAB Function  TreatAsAtomicUnit=on
  i2 : Constant  Value=[1 ,0 ,0]'
  inertial tensor of arm : Constant  Value=[0.012 0 0; 0 0.008 0;0 0 0.019]
  M : Outport
  wires:
  Matrix Multiply3/1 -> Cross Product1/1, Matrix Multiply2/2
  inertial tensor of arm/1 -> Matrix Multiply5/1, Matrix Multiply2/1
  thetadotdot/1 -> Matrix Multiply4/1
  Matrix Multiply4/1 -> Matrix Multiply5/2
  Matrix Multiply5/1 -> Add1/2
  i2/1 -> Matrix Multiply4/2, Matrix Multiply3/2
  arm to body/1(y) -> Matrix Multiply6/1
  Matrix Multiply2/1 -> Cross Product1/2
  Cross Product1/1 -> Add1/1
  Add1/1 -> Matrix Multiply6/2
  thetadot/1 -> Matrix Multiply3/1
  Matrix Multiply6/1 -> M/1
  theta/1 -> arm to body/1(theta)

== system heli/6 DOF VTOL (AEROBLK)/Vehicle dynamics/Arm 3/Prop Froces and moment1 ==
  note: T = Ctx w^2
      | Q = Cd x w^2
  Cd : Inport
  Ct : Inport  Port=2
  omega : Inport  Port=3
  Product{,1..3} (4 alike) : Product
  F : Outport
  M : Outport  Port=2
  wires:
  omega/1 -> Product3/1, Product2/2, Product1/2, Product/2
  Ct/1 -> Product2/1
  Product2/1 -> Product3/2
  Product3/1 -> F/1
  Product/1 -> Product1/1
  Product1/1 -> M/1
  Cd/1 -> Product/1

== system heli/6 DOF VTOL (AEROBLK)/Vehicle dynamics/Arm 3/Subsystem2 ==
  In1 : Inport
  Derivative : Derivative
  Derivative1 : Derivative
  Transfer Fcn (with initial states)1 : simulink_extras/Additional Linear/Transfer Fcn (with initial states)  N=[153.5000]  D="[1  20.06  153.3]"  X0=0
  theta : Outport
  thetadot : Outport  Port=2
  thetadotdot : Outport  Port=3
  wires:
  Derivative/1 -> thetadot/1, Derivative1/1
  Transfer Fcn (with initial states)1/1 -> Derivative/1, theta/1
  Derivative1/1 -> thetadotdot/1
  In1/1 -> Transfer Fcn (with initial states)1/1

== system heli/6 DOF VTOL (AEROBLK)/Vehicle dynamics/Arm 3/Subsystem3 ==
  In1 : Inport
  Derivative2 : Derivative
  Derivative3 : Derivative
  Transfer Fcn (with initial states) : simulink_extras/Additional Linear/Transfer Fcn (with initial states)  N=[153.5000]  D="[1  20.06  153.3]"  X0=0
  phi : Outport
  phidot : Outport  Port=2
  phidotdot : Outport  Port=3
  wires:
  Derivative2/1 -> phidot/1, Derivative3/1
  Transfer Fcn (with initial states)/1 -> Derivative2/1, phi/1
  Derivative3/1 -> phidotdot/1
  In1/1 -> Transfer Fcn (with initial states)/1

== system heli/6 DOF VTOL (AEROBLK)/Vehicle dynamics/Arm 4/Arm dynamics ==
  note: M = I.thetadotdot + thetadot X I.thetadot
      | followed by a conversion to body frame
  theta : Inport
  thetadot : Inport  Port=2
  thetadotdot : Inport  Port=3
  Add1 : Sum
  Cross Product1 : matrix_library/Cross Product
  Matrix Multiply2 : Product  Multiplication=Matrix(*)
  Matrix Multiply3 : Product
  Matrix Multiply4 : Product
  Matrix Multiply5 : Product  Multiplication=Matrix(*)
  Matrix Multiply6 : Product  Multiplication=Matrix(*)
  arm to body : MATLAB Function  TreatAsAtomicUnit=on
  i2 : Constant  Value=[1 ,0 ,0]'
  inertial tensor of arm : Constant  Value=[0.012 0 0; 0 0.008 0;0 0 0.019]
  M : Outport
  wires:
  Matrix Multiply3/1 -> Cross Product1/1, Matrix Multiply2/2
  inertial tensor of arm/1 -> Matrix Multiply5/1, Matrix Multiply2/1
  thetadotdot/1 -> Matrix Multiply4/1
  Matrix Multiply4/1 -> Matrix Multiply5/2
  Matrix Multiply5/1 -> Add1/2
  i2/1 -> Matrix Multiply4/2, Matrix Multiply3/2
  arm to body/1(y) -> Matrix Multiply6/1
  Matrix Multiply2/1 -> Cross Product1/2
  Cross Product1/1 -> Add1/1
  Add1/1 -> Matrix Multiply6/2
  thetadot/1 -> Matrix Multiply3/1
  Matrix Multiply6/1 -> M/1
  theta/1 -> arm to body/1(theta)

== system heli/6 DOF VTOL (AEROBLK)/Vehicle dynamics/Arm 4/Prop Froces and moment1 ==
  note: T = Ctx w^2
      | Q = Cd x w^2
  Cd : Inport
  Ct : Inport  Port=2
  omega : Inport  Port=3
  Product{,1..3} (4 alike) : Product
  F : Outport
  M : Outport  Port=2
  wires:
  omega/1 -> Product3/1, Product2/2, Product1/2, Product/2
  Ct/1 -> Product2/1
  Product2/1 -> Product3/2
  Product3/1 -> F/1
  Product/1 -> Product1/1
  Product1/1 -> M/1
  Cd/1 -> Product/1

== system heli/6 DOF VTOL (AEROBLK)/Vehicle dynamics/Arm 4/Subsystem2 ==
  In1 : Inport
  Derivative : Derivative
  Derivative1 : Derivative
  Transfer Fcn (with initial states)1 : simulink_extras/Additional Linear/Transfer Fcn (with initial states)  N=[153.5000]  D="[1  20.06  153.3]"  X0=0
  theta : Outport
  thetadot : Outport  Port=2
  thetadotdot : Outport  Port=3
  wires:
  Derivative/1 -> thetadot/1, Derivative1/1
  Transfer Fcn (with initial states)1/1 -> Derivative/1, theta/1
  Derivative1/1 -> thetadotdot/1
  In1/1 -> Transfer Fcn (with initial states)1/1

== system heli/6 DOF VTOL (AEROBLK)/Vehicle dynamics/Arm 4/Subsystem3 ==
  In1 : Inport
  Derivative2 : Derivative
  Derivative3 : Derivative
  Transfer Fcn (with initial states) : simulink_extras/Additional Linear/Transfer Fcn (with initial states)  N=[153.5000]  D="[1  20.06  153.3]"  X0=0
  phi : Outport
  phidot : Outport  Port=2
  phidotdot : Outport  Port=3
  wires:
  Derivative2/1 -> phidot/1, Derivative3/1
  Transfer Fcn (with initial states)/1 -> Derivative2/1, phi/1
  Derivative3/1 -> phidotdot/1
  In1/1 -> Transfer Fcn (with initial states)/1

== matlab function heli/6 DOF VTOL (AEROBLK)/Vehicle dynamics/Arm 3/prop to body1 ==
  data: theta input; phi input; y output
function y = fcn(theta, phi)

y = [sin(phi); -sin(theta)*cos(phi); cos(theta)*cos(phi)]; %derived in the literature

== matlab function heli/6 DOF VTOL (AEROBLK)/Vehicle dynamics/Arm 2/prop to body ==
  data: theta input; phi input; y output
function y = fcn(theta, phi)

y = [sin(phi); -sin(theta)*cos(phi); cos(theta)*cos(phi)]; %derived in the literature

== matlab function heli/6 DOF VTOL (AEROBLK)/Vehicle dynamics/Arm 4/Arm dynamics/arm to body ==
  data: theta input; y output
function y = fcn(theta)

theta = -theta; %negating because rotation is from arm to body frame, so angle of rotation will be opposite that of that arm

y = [1 0 0;
    0 cos(theta) -sin(theta);
    0 sin(theta) cos(theta)]; %a rotation about x axis

== matlab function heli/6 DOF VTOL (AEROBLK)/Vehicle dynamics/Arm 4/prop to body1 ==
  data: theta input; phi input; y output
function y = fcn(theta, phi)

y = [sin(phi); -sin(theta)*cos(phi); cos(theta)*cos(phi)]; %derived in the literature

== matlab function heli/Controls (in)/Subsystem/MATLAB Function10 ==
  data: u input; max_out parameter; min_out parameter; max_in parameter; y output; min_in parameter
function y = fcn(u, max_out, min_out, max_in, min_in)

y = (max_out - min_out) / (max_in - min_in) *(u - (min_in + max_in)/2) + (max_out + min_out)/2;

== matlab function heli/Controls (in)/Subsystem/MATLAB Function1 ==
  data: u input; max_out parameter; min_out parameter; max_in parameter; y output; min_in parameter
function y = fcn(u, max_out, min_out, max_in, min_in)

y = (max_out - min_out) / (max_in - min_in) *(u - (min_in + max_in)/2) + (max_out + min_out)/2;

== matlab function heli/Controls (in)/Subsystem/MATLAB Function11 ==
  data: u input; max_out parameter; min_out parameter; max_in parameter; y output; min_in parameter
function y = fcn(u, max_out, min_out, max_in, min_in)

y = (max_out - min_out) / (max_in - min_in) *(u - (min_in + max_in)/2) + (max_out + min_out)/2;

== matlab function heli/6 DOF VTOL (AEROBLK)/Vehicle dynamics/Arm 2/Arm dynamics/arm to body ==
  data: theta input; y output
function y = fcn(theta)

theta = -theta; %negating because rotation is from arm to body frame, so angle of rotation will be opposite that of that arm

y = [1 0 0;
    0 cos(theta) -sin(theta);
    0 sin(theta) cos(theta)]; %a rotation about x axis

== matlab function heli/6 DOF VTOL (AEROBLK)/Vehicle dynamics/Arm 1/prop to body1 ==
  data: theta input; phi input; y output
function y = fcn(theta, phi)

y = [sin(phi); -sin(theta)*cos(phi); cos(theta)*cos(phi)]; %derived in the literature

== matlab function heli/Controls (in)/Subsystem/MATLAB Function12 ==
  data: u input; max_out parameter; min_out parameter; max_in parameter; y output; min_in parameter
function y = fcn(u, max_out, min_out, max_in, min_in)

y = (max_out - min_out) / (max_in - min_in) *(u - (min_in + max_in)/2) + (max_out + min_out)/2;

== matlab function heli/Controls (in)/Subsystem/MATLAB Function9 ==
  data: u input; max_out parameter; min_out parameter; max_in parameter; y output; min_in parameter
function y = fcn(u, max_out, min_out, max_in, min_in)

y = (max_out - min_out) / (max_in - min_in) *(u - (min_in + max_in)/2) + (max_out + min_out)/2;

== matlab function heli/6 DOF VTOL (AEROBLK)/Simulated floor ==
  data: x input; F output; x1 parameter; x2 parameter; thickness parameter; E parameter; A parameter
function F   = wall(x, x1, x2, thickness, E, A)
    [d, direction] = point_to_line_segment_distance(x, x1, x2);
    if d <= thickness
        forceMagnitude = E * (thickness - d)/thickness * A;
        F = forceMagnitude * direction;
    else
        F = [0; 0; 0];
    end
end

function [d, direction] = point_to_line_segment_distance(x, a, b)
    ab = b - a; 
    ax = x(2:3) - a; 
    t = dot(ax, ab) / dot(ab, ab);
    t = max(0, min(1, t));
    closestPoint = a + t * ab;
    normal = [-ab(2); ab(1)];
    if dot(normal, ax) < 0
        normal = -normal;
    end
    direction = normal / norm(normal);
    direction = [0; direction];
    d = norm(x(2:3) - closestPoint);
end

== matlab function heli/Controls (in)/Subsystem/MATLAB Function6 ==
  data: u input; max_out parameter; min_out parameter; max_in parameter; y output; min_in parameter
function y = fcn(u, max_out, min_out, max_in, min_in)

y = (max_out - min_out) / (max_in - min_in) *(u - (min_in + max_in)/2) + (max_out + min_out)/2;

== matlab function heli/Controls (in)/Subsystem/MATLAB Function2 ==
  data: u input; max_out parameter; min_out parameter; max_in parameter; y output; min_in parameter
function y = fcn(u, max_out, min_out, max_in, min_in)

y = (max_out - min_out) / (max_in - min_in) *(u - (min_in + max_in)/2) + (max_out + min_out)/2;

== matlab function heli/Controls (in)/Subsystem/MATLAB Function3 ==
  data: u input; max_out parameter; min_out parameter; max_in parameter; y output; min_in parameter
function y = fcn(u, max_out, min_out, max_in, min_in)

y = (max_out - min_out) / (max_in - min_in) *(u - (min_in + max_in)/2) + (max_out + min_out)/2;

== matlab function heli/Controls (in)/Subsystem/MATLAB Function4 ==
  data: u input; max_out parameter; min_out parameter; max_in parameter; y output; min_in parameter
function y = fcn(u, max_out, min_out, max_in, min_in)

y = (max_out - min_out) / (max_in - min_in) *(u - (min_in + max_in)/2) + (max_out + min_out)/2;

== matlab function heli/Controls (in)/Subsystem/MATLAB Function5 ==
  data: u input; max_out parameter; min_out parameter; max_in parameter; y output; min_in parameter
function y = fcn(u, max_out, min_out, max_in, min_in)

y = (max_out - min_out) / (max_in - min_in) *(u - (min_in + max_in)/2) + (max_out + min_out)/2;

== matlab function heli/Controls (in)/Subsystem/MATLAB Function7 ==
  data: u input; max_out parameter; min_out parameter; max_in parameter; y output; min_in parameter
function y = fcn(u, max_out, min_out, max_in, min_in)

y = (max_out - min_out) / (max_in - min_in) *(u - (min_in + max_in)/2) + (max_out + min_out)/2;

== matlab function heli/Controls (in)/Subsystem/MATLAB Function8 ==
  data: u input; max_out parameter; min_out parameter; max_in parameter; y output; min_in parameter
function y = fcn(u, max_out, min_out, max_in, min_in)

y = (max_out - min_out) / (max_in - min_in) *(u - (min_in + max_in)/2) + (max_out + min_out)/2;

== matlab function heli/6 DOF VTOL (AEROBLK)/Vehicle dynamics/Arm 3/Arm dynamics/arm to body ==
  data: theta input; y output
function y = fcn(theta)

theta = -theta; %negating because rotation is from arm to body frame, so angle of rotation will be opposite that of that arm

y = [1 0 0;
    0 cos(theta) -sin(theta);
    0 sin(theta) cos(theta)]; %a rotation about x axis

== matlab function heli/6 DOF VTOL (AEROBLK)/Vehicle dynamics/Arm 1/Arm dynamics/arm to body ==
  data: theta input; y output
function y = fcn(theta)

theta = -theta; %negating because rotation is from arm to body frame, so angle of rotation will be opposite that of that arm

y = [1 0 0;
    0 cos(theta) -sin(theta);
    0 sin(theta) cos(theta)]; %a rotation about x axis
